simulink model "ddc_bpm_476_066"  (Simulink 7.8)
settings: Solver=ode45  StartTime=0.0  StopTime=2e-3  RelTol=1e-3
undefined symbols (not defined in the file): decim_factor_poly_35, dt_sim, frev_476, Fs_adc, n_ch, n_ovs, R_fofb, R_sec, R_sec_cfir, R_sec_pfir, xlipgetpartsetting
libraries: xbsIndex_r4 x1491, simulink x7
(part 1 of 12)
settings Model: Creator=lucas.russo  LastModifiedBy=lucas.russo
settings HardwareCC: ProdHWDeviceType=ASIC/FPGA->ASIC/FPGA  TargetIntDivRoundTo=Zero  TargetEndianess=LittleEndian  TargetHWDeviceType=MATLAB Host  ProdEqTarget=off

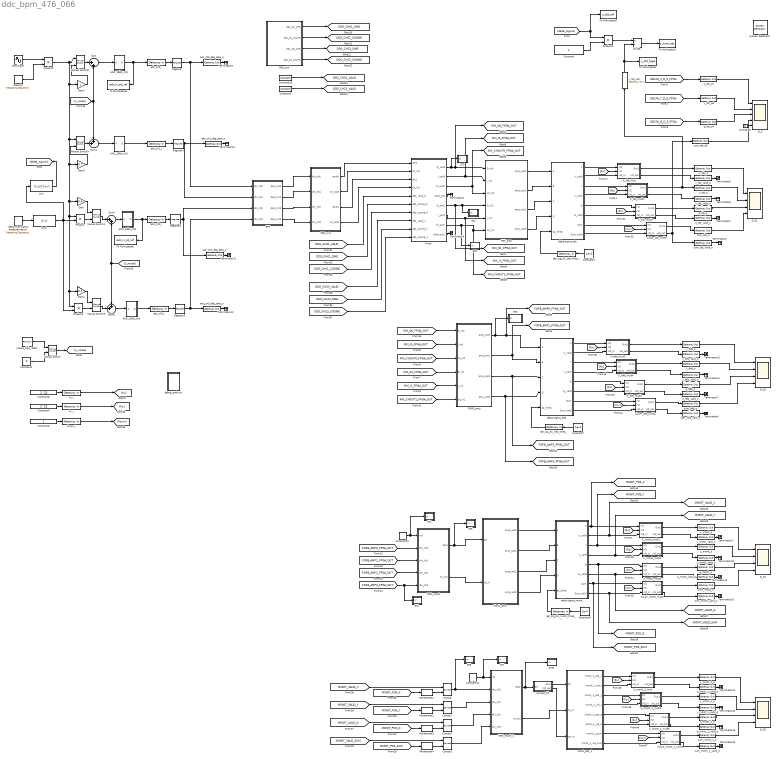
== system ddc_bpm_476_066 ==
  " System Generator" : xbsIndex_r4/ System Generator  Tag=genX  xilinxfamily=artix7  part=xc7a200t  speed=-1  package=ffg1156  synthesis_tool=XST  clock_wrapper=Clock Enables  directory=./netlist_ddc_bpm_476_066_artix7  proj_type=Project Navigator  Synth_file=XST Defaults  Impl_file=ISE Defaults  testbench=off  simulink_period=1/Fs_adc/n_ovs  sysclk_period=1/Fs_adc/n_ovs*1e9  dcm_input_clock_period=10  incr_netlist=off  trim_vbits=Everywhere in SubSystem  dbl_ovrd=According to Block Masks  core_generation=According to Block Masks  run_coregen=off  deprecated_control=off  eval_field=0  block_type=sysgen
  ADC_16bit_ch0 : Subsystem
  ADC_16bit_ch1 : Subsystem
  ADC_16bit_ch2 : Subsystem
  ADC_16bit_ch3 : Subsystem
  BPF : Subsystem
  Concat{,1..3} (4 alike) : xbsIndex_r4/Concat  num_inputs=2  dbl_ovrd=off  block_type=concat
  Constant : Constant
  Constant1 : Constant  Value=1e-4  OutDataTypeStr=fixdt(1,26,22)
  Constant10 : xbsIndex_r4/Constant  const=0  gui_display_data_type=Boolean  arith_type=Boolean  n_bits=16  bin_pt=14  preci_type=Single  exp_width=8  frac_width=24  explicit_period=on  period=(1/Fs_adc*R_fofb)/n_ovs/2  equ=P=C  opselect=C  inp2=PCIN>>17  opr=+  inp1=P  carry=CIN  dbl_ovrd=off  block_type=constant
  Constant11 : xbsIndex_r4/Constant  const=0  gui_display_data_type=Boolean  arith_type=Boolean  n_bits=16  bin_pt=14  preci_type=Single  exp_width=8  frac_width=24  explicit_period=on  period=(1/Fs_adc*R_fofb*R_sec*R_sec_cfir*R_sec_pfir)/n_ovs/2  equ=P=C  opselect=C  inp2=PCIN>>17  opr=+  inp1=P  carry=CIN  dbl_ovrd=off  block_type=constant
  Constant15 : xbsIndex_r4/Constant  const=1  gui_display_data_type=Boolean  arith_type=Boolean  n_bits=24  bin_pt=22  preci_type=Single  exp_width=8  frac_width=24  explicit_period=on  period=1/Fs_adc/n_ovs  equ=P=C  opselect=C  inp2=PCIN>>17  opr=+  inp1=P  carry=CIN  dbl_ovrd=off  block_type=constant
  Constant2 : Constant  Value=0  SampleTime=0
  Constant3 : xbsIndex_r4/Constant  const=1  gui_display_data_type=Boolean  arith_type=Boolean  n_bits=24  bin_pt=22  preci_type=Single  exp_width=8  frac_width=24  explicit_period=on  period=1/Fs_adc/n_ovs  equ=P=C  opselect=C  inp2=PCIN>>17  opr=+  inp1=P  carry=CIN  dbl_ovrd=off  block_type=constant
  Constant4 : Constant  Value=2^23
  Constant5 : Constant  Value=0
  Constant6 : Constant
  Constant7 : Constant  Value=1e-4  OutDataTypeStr=fixdt(1,26,22)
  Constant8 : Constant  Value=2^23
  Constant9 : Constant  Value=1e-4  OutDataTypeStr=fixdt(1,26,22)
  DDS_sub : Subsystem
  D_S : Scope  NumInputPorts=5
      settings: TimeRange=0.0004  YMin=-1~0~10~0~0  YMax=1~0.00025~100~2.5~1  SaveName=ScopeData7  MaxDataPoints=1000000  SampleInput=on
  D_S{1,3..5} (4 alike) : Scope  NumInputPorts=4
      D_S1 settings: TimeRange=0.0003  YMin=-1~-1~-1~0.414326  YMax=1~1~1~0.414329  SaveName=ScopeData6  MaxDataPoints=1000000  SampleInput=on
      D_S3 settings: TimeRange=0.0003  YMin=-1~-1~-1~0.0190031  YMax=1~1~1~0.0210035  SaveName=ScopeData2  MaxDataPoints=1000000  SampleInput=on
      D_S4 settings: TimeRange=0.0003  YMin=-1~-1~-1~0.0190031  YMax=1~1~1~0.0210035  SaveName=ScopeData3  MaxDataPoints=1000000  SampleInput=on
      D_S5 settings: TimeRange=0.0003  YMin=-1~-1~-1~0.0190031  YMax=1~1~1~0.0210035  SaveName=ScopeData20  MaxDataPoints=1000000  SampleInput=on
  Divide : Product  Inputs=*/
  FOFB_amp : Subsystem
  Fcn : Fcn  Expr=(1-u)/(1+u)
  Fcn1 : Fcn  Expr=(1-u)
  Gain : Gain  Gain=0.4
  Gain2 : Gain
  Gain3 : Gain  Gain=0.7
  Gain4 : Gain  Gain=0.1
  K_fofb_mult3 : Subsystem
  K_fofb_mult4 : Subsystem
  K_fofb_mult5 : Subsystem
  K_monit_1_mult : Subsystem
  K_monit_1_mult2 : Subsystem
  K_monit_1_mult6 : Subsystem
  K_monit_mult3 : Subsystem
  K_monit_mult4 : Subsystem
  K_monit_mult5 : Subsystem
  K_tbt_mult : Subsystem
  K_tbt_mult1 : Subsystem
  K_tbt_mult2 : Subsystem
  Ksum_fofb_mult4 : Subsystem
  Ksum_i : xbsIndex_r4/Gateway In  gui_display_data_type=Fixed-point  arith_type="Signed  (2's comp)"  n_bits=25  bin_pt=23  preci_type=Single  exp_width=8  frac_width=24  quantization=Truncate  overflow=Flag as error  period=1/Fs_adc  dbl_ovrd=off  timing_constraint=Data Rate  locs_specified=off  LOCs={}  inherit_from_input=off  UseAsADC=off  ADCChannel='1'  hdl_port=on  block_type=gatewayin
      settings: infoedit="Gateway in block.  Converts inputs of type Simulink integer, single, double and fixed point to  Xilinx fixed-point or floating-point data type.<br><br>Hardware notes:  In hardware these blocks become top level input ports."
  Ksum_monit_1_mult1 : Subsystem
  Ksum_monit_mult2 : Subsystem
  Ksum_tbt_mult3 : Subsystem
  Kx_i : xbsIndex_r4/Gateway In  gui_display_data_type=Fixed-point  arith_type="Signed  (2's comp)"  n_bits=25  bin_pt=0  preci_type=Single  exp_width=8  frac_width=24  quantization=Truncate  overflow=Flag as error  period=1/Fs_adc  dbl_ovrd=off  timing_constraint=Data Rate  locs_specified=off  LOCs={}  inherit_from_input=off  UseAsADC=off  ADCChannel='1'  hdl_port=on  block_type=gatewayin
      settings: infoedit="Gateway in block.  Converts inputs of type Simulink integer, single, double and fixed point to  Xilinx fixed-point or floating-point data type.<br><br>Hardware notes:  In hardware these blocks become top level input ports."
  Ky_i : xbsIndex_r4/Gateway In  gui_display_data_type=Fixed-point  arith_type="Signed  (2's comp)"  n_bits=25  bin_pt=0  preci_type=Single  exp_width=8  frac_width=24  quantization=Truncate  overflow=Flag as error  period=1/Fs_adc  dbl_ovrd=off  timing_constraint=Data Rate  locs_specified=off  LOCs={}  inherit_from_input=off  UseAsADC=off  ADCChannel='1'  hdl_port=on  block_type=gatewayin
      settings: infoedit="Gateway in block.  Converts inputs of type Simulink integer, single, double and fixed point to  Xilinx fixed-point or floating-point data type.<br><br>Hardware notes:  In hardware these blocks become top level input ports."
  Manual Switch : simulink/Signal Routing/Manual Switch  sw=0  action=0  varsize=off
  Manual Switch2 : simulink/Signal Routing/Manual Switch  sw=0  action=0  varsize=off
  Manual Switch3 : simulink/Signal Routing/Manual Switch  sw=0  action=0  varsize=off
  Manual Switch4 : simulink/Signal Routing/Manual Switch  sw=1  action=0  varsize=off
  Manual Switch5 : simulink/Signal Routing/Manual Switch  sw=1  action=0  varsize=off
  Mixer : Subsystem
  Monit_amp : Subsystem
  Product{,1..3} (4 alike) : Product  RndMeth=Zero
  Register{,1..3} (4 alike) : xbsIndex_r4/Register  init=0  rst=off  en=off  dbl_ovrd=off  block_type=register
  Reinterpret{1..4} (4 alike) : xbsIndex_r4/Reinterpret  force_arith_type=on  arith_type=Unsigned  force_bin_pt=on  bin_pt=0  block_type=reinterpret
  ST1 : Subsystem
  ST10 : Subsystem
  ST2 : Subsystem
  ST3 : Subsystem
  ST4 : Subsystem
  ST5 : Subsystem
  ST6 : Subsystem
  ST7 : Subsystem
  ST8 : Subsystem
  ST9 : Subsystem
  Sine Wave : Sin  Frequency=2*pi*frev_476  SampleTime=0
  Sum : Sum  Inputs=|++
  Sum1 : Sum  Inputs=++|
  Sum2 : Sum  Inputs=|++
  Sum3 : Sum  Inputs=++|
  TBT_amp : Subsystem
  TDM_mix : Subsystem
  TDM_monit : Subsystem
  TDM_monit_1 : Subsystem
  Terminator{1..22} (22 alike) : Terminator
  To Workspace1 : ToWorkspace  VariableName=y_tbt_fpga  SampleTime=-1  SaveFormat=Structure With Time
  To Workspace2 : ToWorkspace  VariableName=y_error_tbt  SampleTime=-1  SaveFormat=Structure With Time
  To Workspace3 : ToWorkspace  VariableName=y_tbt_ref  SampleTime=-1  SaveFormat=Structure With Time
  To Workspace4 : ToWorkspace  VariableName=adc_in_ab_ref  SampleTime=-1  SaveFormat=Structure With Time
  To Workspace5 : ToWorkspace  VariableName=adc_in_cd_ref  SampleTime=-1  SaveFormat=Structure With Time
  adc_ch0_dbg_data_o : xbsIndex_r4/Gateway Out  inherit_from_input=on  hdl_port=on  timing_constraint=Data Rate  locs_specified=off  LOCs={}  UseAsDAC=off  DACChannel='1'  block_type=gatewayout
      settings: infoedit="Gateway out block.  Converts Xilinx fixed-point or floating-point type inputs into ouputs of type Simulink integer, single, double, or fixed point.<br><br>Hardware notes:  In hardware these blocks become top level output ports or are discarded, depending on how they are configured."
  adc_ch0_i : xbsIndex_r4/Gateway In  gui_display_data_type=Fixed-point  arith_type="Signed  (2's comp)"  n_bits=16  bin_pt=15  preci_type=Single  exp_width=8  frac_width=24  quantization=Truncate  overflow=Flag as error  period=1/Fs_adc  dbl_ovrd=off  timing_constraint=None  locs_specified=off  LOCs={}  inherit_from_input=off  UseAsADC=off  ADCChannel='1'  hdl_port=on  block_type=gatewayin
      settings: infoedit="Gateway in block.  Converts inputs of type Simulink integer, single, double and fixed point to  Xilinx fixed-point or floating-point data type.<br><br>Hardware notes:  In hardware these blocks become top level input ports."
  adc_ch1_dbg_data_o : xbsIndex_r4/Gateway Out  inherit_from_input=on  hdl_port=on  timing_constraint=Data Rate  locs_specified=off  LOCs={}  UseAsDAC=off  DACChannel='1'  block_type=gatewayout
      settings: infoedit="Gateway out block.  Converts Xilinx fixed-point or floating-point type inputs into ouputs of type Simulink integer, single, double, or fixed point.<br><br>Hardware notes:  In hardware these blocks become top level output ports or are discarded, depending on how they are configured."
  adc_ch1_i : xbsIndex_r4/Gateway In  gui_display_data_type=Fixed-point  arith_type="Signed  (2's comp)"  n_bits=16  bin_pt=15  preci_type=Single  exp_width=8  frac_width=24  quantization=Truncate  overflow=Flag as error  period=1/Fs_adc  dbl_ovrd=off  timing_constraint=None  locs_specified=off  LOCs={}  inherit_from_input=off  UseAsADC=off  ADCChannel='1'  hdl_port=on  block_type=gatewayin
      settings: infoedit="Gateway in block.  Converts inputs of type Simulink integer, single, double and fixed point to  Xilinx fixed-point or floating-point data type.<br><br>Hardware notes:  In hardware these blocks become top level input ports."
  adc_ch2_dbg_data_o : xbsIndex_r4/Gateway Out  inherit_from_input=on  hdl_port=on  timing_constraint=Data Rate  locs_specified=off  LOCs={}  UseAsDAC=off  DACChannel='1'  block_type=gatewayout
      settings: infoedit="Gateway out block.  Converts Xilinx fixed-point or floating-point type inputs into ouputs of type Simulink integer, single, double, or fixed point.<br><br>Hardware notes:  In hardware these blocks become top level output ports or are discarded, depending on how they are configured."
  adc_ch2_i : xbsIndex_r4/Gateway In  gui_display_data_type=Fixed-point  arith_type="Signed  (2's comp)"  n_bits=16  bin_pt=15  preci_type=Single  exp_width=8  frac_width=24  quantization=Truncate  overflow=Flag as error  period=1/Fs_adc  dbl_ovrd=off  timing_constraint=None  locs_specified=off  LOCs={}  inherit_from_input=off  UseAsADC=off  ADCChannel='1'  hdl_port=on  block_type=gatewayin
      settings: infoedit="Gateway in block.  Converts inputs of type Simulink integer, single, double and fixed point to  Xilinx fixed-point or floating-point data type.<br><br>Hardware notes:  In hardware these blocks become top level input ports."
  adc_ch3_dbg_data_o : xbsIndex_r4/Gateway Out  inherit_from_input=on  hdl_port=on  timing_constraint=Data Rate  locs_specified=off  LOCs={}  UseAsDAC=off  DACChannel='1'  block_type=gatewayout
      settings: infoedit="Gateway out block.  Converts Xilinx fixed-point or floating-point type inputs into ouputs of type Simulink integer, single, double, or fixed point.<br><br>Hardware notes:  In hardware these blocks become top level output ports or are discarded, depending on how they are configured."
  adc_ch3_i : xbsIndex_r4/Gateway In  gui_display_data_type=Fixed-point  arith_type="Signed  (2's comp)"  n_bits=16  bin_pt=15  preci_type=Single  exp_width=8  frac_width=24  quantization=Truncate  overflow=Flag as error  period=1/Fs_adc  dbl_ovrd=off  timing_constraint=None  locs_specified=off  LOCs={}  inherit_from_input=off  UseAsADC=off  ADCChannel='1'  hdl_port=on  block_type=gatewayin
      settings: infoedit="Gateway in block.  Converts inputs of type Simulink integer, single, double and fixed point to  Xilinx fixed-point or floating-point data type.<br><br>Hardware notes:  In hardware these blocks become top level input ports."
  convert_filt : Subsystem
  debug_analysis : Subsystem
  del_sig_div_fofb_thres_i : xbsIndex_r4/Gateway In  gui_display_data_type=Fixed-point  arith_type="Signed  (2's comp)"  n_bits=26  bin_pt=22  preci_type=Single  exp_width=8  frac_width=24  quantization=Truncate  overflow=Flag as error  period=1/Fs_adc  dbl_ovrd=off  timing_constraint=Data Rate  locs_specified=off  LOCs={}  inherit_from_input=off  UseAsADC=off  ADCChannel='1'  hdl_port=on  block_type=gatewayin
      settings: infoedit="Gateway in block.  Converts inputs of type Simulink integer, single, double and fixed point to  Xilinx fixed-point or floating-point data type.<br><br>Hardware notes:  In hardware these blocks become top level input ports."
  del_sig_div_monit_thres_i : xbsIndex_r4/Gateway In  gui_display_data_type=Fixed-point  arith_type="Signed  (2's comp)"  n_bits=26  bin_pt=22  preci_type=Single  exp_width=8  frac_width=24  quantization=Truncate  overflow=Flag as error  period=1/Fs_adc  dbl_ovrd=off  timing_constraint=Data Rate  locs_specified=off  LOCs={}  inherit_from_input=off  UseAsADC=off  ADCChannel='1'  hdl_port=on  block_type=gatewayin
      settings: infoedit="Gateway in block.  Converts inputs of type Simulink integer, single, double and fixed point to  Xilinx fixed-point or floating-point data type.<br><br>Hardware notes:  In hardware these blocks become top level input ports."
  del_sig_div_tbt_thres_i : xbsIndex_r4/Gateway In  gui_display_data_type=Fixed-point  arith_type="Signed  (2's comp)"  n_bits=26  bin_pt=22  preci_type=Single  exp_width=8  frac_width=24  quantization=Truncate  overflow=Flag as error  period=1/Fs_adc  dbl_ovrd=off  timing_constraint=Data Rate  locs_specified=off  LOCs={}  inherit_from_input=off  UseAsADC=off  ADCChannel='1'  hdl_port=on  block_type=gatewayin
      settings: infoedit="Gateway in block.  Converts inputs of type Simulink integer, single, double and fixed point to  Xilinx fixed-point or floating-point data type.<br><br>Hardware notes:  In hardware these blocks become top level input ports."
  delta-over-sigma expected result : simulink/Sources/Repeating Sequence  rep_seq_t=[0 0.25e-4 0.25e-4 0.5e-4 0.5e-4 0.75e-4 0.75e-4 1e-4]  rep_seq_y=0.5 * [1 1 1 1 1 1 1 1]
  delta-sigma_fofb : Subsystem
  delta-sigma_monit : Subsystem
  delta-sigma_tbt : Subsystem
  intensity : simulink/Sources/Repeating Sequence  rep_seq_t=[0 1e-4 1e-4 2e-4 2e-4 3e-4 3e-4 4e-4]  rep_seq_y=[1 1 0.1 0.1 0.01 0.01 0.001 0.001]
  monit_pos_1 : Subsystem
  q_fofb_o : xbsIndex_r4/Gateway Out  inherit_from_input=on  hdl_port=on  timing_constraint=None  locs_specified=off  LOCs={}  UseAsDAC=off  DACChannel='1'  block_type=gatewayout
      settings: infoedit="Gateway out block.  Converts Xilinx fixed-point or floating-point type inputs into ouputs of type Simulink integer, single, double, or fixed point.<br><br>Hardware notes:  In hardware these blocks become top level output ports or are discarded, depending on how they are configured."
  q_fofb_valid_o : xbsIndex_r4/Gateway Out  inherit_from_input=on  hdl_port=on  timing_constraint=Data Rate  locs_specified=off  LOCs={}  UseAsDAC=off  DACChannel='1'  block_type=gatewayout
      settings: infoedit="Gateway out block.  Converts Xilinx fixed-point or floating-point type inputs into ouputs of type Simulink integer, single, double, or fixed point.<br><br>Hardware notes:  In hardware these blocks become top level output ports or are discarded, depending on how they are configured."
  q_monit_1_o : xbsIndex_r4/Gateway Out  inherit_from_input=on  hdl_port=on  timing_constraint=None  locs_specified=off  LOCs={}  UseAsDAC=off  DACChannel='1'  block_type=gatewayout
      settings: infoedit="Gateway out block.  Converts Xilinx fixed-point or floating-point type inputs into ouputs of type Simulink integer, single, double, or fixed point.<br><br>Hardware notes:  In hardware these blocks become top level output ports or are discarded, depending on how they are configured."
  q_monit_1_valid_o : xbsIndex_r4/Gateway Out  inherit_from_input=on  hdl_port=on  timing_constraint=Data Rate  locs_specified=off  LOCs={}  UseAsDAC=off  DACChannel='1'  block_type=gatewayout
      settings: infoedit="Gateway out block.  Converts Xilinx fixed-point or floating-point type inputs into ouputs of type Simulink integer, single, double, or fixed point.<br><br>Hardware notes:  In hardware these blocks become top level output ports or are discarded, depending on how they are configured."
  q_monit_o : xbsIndex_r4/Gateway Out  inherit_from_input=on  hdl_port=on  timing_constraint=None  locs_specified=off  LOCs={}  UseAsDAC=off  DACChannel='1'  block_type=gatewayout
      settings: infoedit="Gateway out block.  Converts Xilinx fixed-point or floating-point type inputs into ouputs of type Simulink integer, single, double, or fixed point.<br><br>Hardware notes:  In hardware these blocks become top level output ports or are discarded, depending on how they are configured."
  q_monit_valid_o : xbsIndex_r4/Gateway Out  inherit_from_input=on  hdl_port=on  timing_constraint=Data Rate  locs_specified=off  LOCs={}  UseAsDAC=off  DACChannel='1'  block_type=gatewayout
      settings: infoedit="Gateway out block.  Converts Xilinx fixed-point or floating-point type inputs into ouputs of type Simulink integer, single, double, or fixed point.<br><br>Hardware notes:  In hardware these blocks become top level output ports or are discarded, depending on how they are configured."
  q_tbt_o : xbsIndex_r4/Gateway Out  inherit_from_input=on  hdl_port=on  timing_constraint=Data Rate  locs_specified=off  LOCs={}  UseAsDAC=off  DACChannel='1'  block_type=gatewayout
      settings: infoedit="Gateway out block.  Converts Xilinx fixed-point or floating-point type inputs into ouputs of type Simulink integer, single, double, or fixed point.<br><br>Hardware notes:  In hardware these blocks become top level output ports or are discarded, depending on how they are configured."
  q_tbt_o4 : xbsIndex_r4/Gateway Out  inherit_from_input=on  hdl_port=off  timing_constraint=None  locs_specified=off  LOCs={}  UseAsDAC=off  DACChannel='1'  block_type=gatewayout
      settings: infoedit="Gateway out block.  Converts Xilinx fixed-point or floating-point type inputs into ouputs of type Simulink integer, single, double, or fixed point.<br><br>Hardware notes:  In hardware these blocks become top level output ports or are discarded, depending on how they are configured."
  q_tbt_valid_o : xbsIndex_r4/Gateway Out  inherit_from_input=on  hdl_port=on  timing_constraint=Data Rate  locs_specified=off  LOCs={}  UseAsDAC=off  DACChannel='1'  block_type=gatewayout
      settings: infoedit="Gateway out block.  Converts Xilinx fixed-point or floating-point type inputs into ouputs of type Simulink integer, single, double, or fixed point.<br><br>Hardware notes:  In hardware these blocks become top level output ports or are discarded, depending on how they are configured."
  sum_fofb_o : xbsIndex_r4/Gateway Out  inherit_from_input=on  hdl_port=on  timing_constraint=None  locs_specified=off  LOCs={}  UseAsDAC=off  DACChannel='1'  block_type=gatewayout
      settings: infoedit="Gateway out block.  Converts Xilinx fixed-point or floating-point type inputs into ouputs of type Simulink integer, single, double, or fixed point.<br><br>Hardware notes:  In hardware these blocks become top level output ports or are discarded, depending on how they are configured."
  sum_fofb_valid_o : xbsIndex_r4/Gateway Out  inherit_from_input=on  hdl_port=on  timing_constraint=Data Rate  locs_specified=off  LOCs={}  UseAsDAC=off  DACChannel='1'  block_type=gatewayout
      settings: infoedit="Gateway out block.  Converts Xilinx fixed-point or floating-point type inputs into ouputs of type Simulink integer, single, double, or fixed point.<br><br>Hardware notes:  In hardware these blocks become top level output ports or are discarded, depending on how they are configured."
  sum_monit_1_o : xbsIndex_r4/Gateway Out  inherit_from_input=on  hdl_port=on  timing_constraint=None  locs_specified=off  LOCs={}  UseAsDAC=off  DACChannel='1'  block_type=gatewayout
      settings: infoedit="Gateway out block.  Converts Xilinx fixed-point or floating-point type inputs into ouputs of type Simulink integer, single, double, or fixed point.<br><br>Hardware notes:  In hardware these blocks become top level output ports or are discarded, depending on how they are configured."
  sum_monit_1_valid_o : xbsIndex_r4/Gateway Out  inherit_from_input=on  hdl_port=on  timing_constraint=Data Rate  locs_specified=off  LOCs={}  UseAsDAC=off  DACChannel='1'  block_type=gatewayout
      settings: infoedit="Gateway out block.  Converts Xilinx fixed-point or floating-point type inputs into ouputs of type Simulink integer, single, double, or fixed point.<br><br>Hardware notes:  In hardware these blocks become top level output ports or are discarded, depending on how they are configured."
  sum_monit_o : xbsIndex_r4/Gateway Out  inherit_from_input=on  hdl_port=on  timing_constraint=None  locs_specified=off  LOCs={}  UseAsDAC=off  DACChannel='1'  block_type=gatewayout
      settings: infoedit="Gateway out block.  Converts Xilinx fixed-point or floating-point type inputs into ouputs of type Simulink integer, single, double, or fixed point.<br><br>Hardware notes:  In hardware these blocks become top level output ports or are discarded, depending on how they are configured."
  sum_monit_valid_o : xbsIndex_r4/Gateway Out  inherit_from_input=on  hdl_port=on  timing_constraint=Data Rate  locs_specified=off  LOCs={}  UseAsDAC=off  DACChannel='1'  block_type=gatewayout
      settings: infoedit="Gateway out block.  Converts Xilinx fixed-point or floating-point type inputs into ouputs of type Simulink integer, single, double, or fixed point.<br><br>Hardware notes:  In hardware these blocks become top level output ports or are discarded, depending on how they are configured."
  sum_tbt_o : xbsIndex_r4/Gateway Out  inherit_from_input=on  hdl_port=on  timing_constraint=Data Rate  locs_specified=off  LOCs={}  UseAsDAC=off  DACChannel='1'  block_type=gatewayout
      settings: infoedit="Gateway out block.  Converts Xilinx fixed-point or floating-point type inputs into ouputs of type Simulink integer, single, double, or fixed point.<br><br>Hardware notes:  In hardware these blocks become top level output ports or are discarded, depending on how they are configured."
  sum_tbt_o5 : xbsIndex_r4/Gateway Out  inherit_from_input=on  hdl_port=off  timing_constraint=None  locs_specified=off  LOCs={}  UseAsDAC=off  DACChannel='1'  block_type=gatewayout
      settings: infoedit="Gateway out block.  Converts Xilinx fixed-point or floating-point type inputs into ouputs of type Simulink integer, single, double, or fixed point.<br><br>Hardware notes:  In hardware these blocks become top level output ports or are discarded, depending on how they are configured."
  sum_tbt_valid_o : xbsIndex_r4/Gateway Out  inherit_from_input=on  hdl_port=on  timing_constraint=Data Rate  locs_specified=off  LOCs={}  UseAsDAC=off  DACChannel='1'  block_type=gatewayout
      settings: infoedit="Gateway out block.  Converts Xilinx fixed-point or floating-point type inputs into ouputs of type Simulink integer, single, double, or fixed point.<br><br>Hardware notes:  In hardware these blocks become top level output ports or are discarded, depending on how they are configured."
  unoise_1lsb_ 16bit : UniformRandomNumber  Minimum=-0.5*(2/2^16)  Maximum=0.5*(2/2^16)  Seed=49728613  SampleTime=0
  x_fofb_o : xbsIndex_r4/Gateway Out  inherit_from_input=on  hdl_port=on  timing_constraint=None  locs_specified=off  LOCs={}  UseAsDAC=off  DACChannel='1'  block_type=gatewayout
      settings: infoedit="Gateway out block.  Converts Xilinx fixed-point or floating-point type inputs into ouputs of type Simulink integer, single, double, or fixed point.<br><br>Hardware notes:  In hardware these blocks become top level output ports or are discarded, depending on how they are configured."
  x_fofb_valid_o : xbsIndex_r4/Gateway Out  inherit_from_input=on  hdl_port=on  timing_constraint=Data Rate  locs_specified=off  LOCs={}  UseAsDAC=off  DACChannel='1'  block_type=gatewayout
      settings: infoedit="Gateway out block.  Converts Xilinx fixed-point or floating-point type inputs into ouputs of type Simulink integer, single, double, or fixed point.<br><br>Hardware notes:  In hardware these blocks become top level output ports or are discarded, depending on how they are configured."
  x_monit_1_o : xbsIndex_r4/Gateway Out  inherit_from_input=on  hdl_port=on  timing_constraint=None  locs_specified=off  LOCs={}  UseAsDAC=off  DACChannel='1'  block_type=gatewayout
      settings: infoedit="Gateway out block.  Converts Xilinx fixed-point or floating-point type inputs into ouputs of type Simulink integer, single, double, or fixed point.<br><br>Hardware notes:  In hardware these blocks become top level output ports or are discarded, depending on how they are configured."
  x_monit_1_valid_o : xbsIndex_r4/Gateway Out  inherit_from_input=on  hdl_port=on  timing_constraint=Data Rate  locs_specified=off  LOCs={}  UseAsDAC=off  DACChannel='1'  block_type=gatewayout
      settings: infoedit="Gateway out block.  Converts Xilinx fixed-point or floating-point type inputs into ouputs of type Simulink integer, single, double, or fixed point.<br><br>Hardware notes:  In hardware these blocks become top level output ports or are discarded, depending on how they are configured."
  x_monit_o : xbsIndex_r4/Gateway Out  inherit_from_input=on  hdl_port=on  timing_constraint=None  locs_specified=off  LOCs={}  UseAsDAC=off  DACChannel='1'  block_type=gatewayout
      settings: infoedit="Gateway out block.  Converts Xilinx fixed-point or floating-point type inputs into ouputs of type Simulink integer, single, double, or fixed point.<br><br>Hardware notes:  In hardware these blocks become top level output ports or are discarded, depending on how they are configured."
  x_monit_valid_o : xbsIndex_r4/Gateway Out  inherit_from_input=on  hdl_port=on  timing_constraint=Data Rate  locs_specified=off  LOCs={}  UseAsDAC=off  DACChannel='1'  block_type=gatewayout
      settings: infoedit="Gateway out block.  Converts Xilinx fixed-point or floating-point type inputs into ouputs of type Simulink integer, single, double, or fixed point.<br><br>Hardware notes:  In hardware these blocks become top level output ports or are discarded, depending on how they are configured."
  x_tbt_o : xbsIndex_r4/Gateway Out  inherit_from_input=on  hdl_port=on  timing_constraint=Data Rate  locs_specified=off  LOCs={}  UseAsDAC=off  DACChannel='1'  block_type=gatewayout
      settings: infoedit="Gateway out block.  Converts Xilinx fixed-point or floating-point type inputs into ouputs of type Simulink integer, single, double, or fixed point.<br><br>Hardware notes:  In hardware these blocks become top level output ports or are discarded, depending on how they are configured."
  x_tbt_o1 : xbsIndex_r4/Gateway Out  inherit_from_input=on  hdl_port=off  timing_constraint=None  locs_specified=off  LOCs={}  UseAsDAC=off  DACChannel='1'  block_type=gatewayout
      settings: infoedit="Gateway out block.  Converts Xilinx fixed-point or floating-point type inputs into ouputs of type Simulink integer, single, double, or fixed point.<br><br>Hardware notes:  In hardware these blocks become top level output ports or are discarded, depending on how they are configured."
  x_tbt_valid_o : xbsIndex_r4/Gateway Out  inherit_from_input=on  hdl_port=on  timing_constraint=Data Rate  locs_specified=off  LOCs={}  UseAsDAC=off  DACChannel='1'  block_type=gatewayout
      settings: infoedit="Gateway out block.  Converts Xilinx fixed-point or floating-point type inputs into ouputs of type Simulink integer, single, double, or fixed point.<br><br>Hardware notes:  In hardware these blocks become top level output ports or are discarded, depending on how they are configured."
  y_fofb_o : xbsIndex_r4/Gateway Out  inherit_from_input=on  hdl_port=on  timing_constraint=None  locs_specified=off  LOCs={}  UseAsDAC=off  DACChannel='1'  block_type=gatewayout
      settings: infoedit="Gateway out block.  Converts Xilinx fixed-point or floating-point type inputs into ouputs of type Simulink integer, single, double, or fixed point.<br><br>Hardware notes:  In hardware these blocks become top level output ports or are discarded, depending on how they are configured."
  y_fofb_valid_o : xbsIndex_r4/Gateway Out  inherit_from_input=on  hdl_port=on  timing_constraint=Data Rate  locs_specified=off  LOCs={}  UseAsDAC=off  DACChannel='1'  block_type=gatewayout
      settings: infoedit="Gateway out block.  Converts Xilinx fixed-point or floating-point type inputs into ouputs of type Simulink integer, single, double, or fixed point.<br><br>Hardware notes:  In hardware these blocks become top level output ports or are discarded, depending on how they are configured."
  y_monit_1_o : xbsIndex_r4/Gateway Out  inherit_from_input=on  hdl_port=on  timing_constraint=None  locs_specified=off  LOCs={}  UseAsDAC=off  DACChannel='1'  block_type=gatewayout
      settings: infoedit="Gateway out block.  Converts Xilinx fixed-point or floating-point type inputs into ouputs of type Simulink integer, single, double, or fixed point.<br><br>Hardware notes:  In hardware these blocks become top level output ports or are discarded, depending on how they are configured."
  y_monit_1_valid_o : xbsIndex_r4/Gateway Out  inherit_from_input=on  hdl_port=on  timing_constraint=Data Rate  locs_specified=off  LOCs={}  UseAsDAC=off  DACChannel='1'  block_type=gatewayout
      settings: infoedit="Gateway out block.  Converts Xilinx fixed-point or floating-point type inputs into ouputs of type Simulink integer, single, double, or fixed point.<br><br>Hardware notes:  In hardware these blocks become top level output ports or are discarded, depending on how they are configured."
  y_monit_o : xbsIndex_r4/Gateway Out  inherit_from_input=on  hdl_port=on  timing_constraint=None  locs_specified=off  LOCs={}  UseAsDAC=off  DACChannel='1'  block_type=gatewayout
      settings: infoedit="Gateway out block.  Converts Xilinx fixed-point or floating-point type inputs into ouputs of type Simulink integer, single, double, or fixed point.<br><br>Hardware notes:  In hardware these blocks become top level output ports or are discarded, depending on how they are configured."
  y_monit_valid_o : xbsIndex_r4/Gateway Out  inherit_from_input=on  hdl_port=on  timing_constraint=Data Rate  locs_specified=off  LOCs={}  UseAsDAC=off  DACChannel='1'  block_type=gatewayout
      settings: infoedit="Gateway out block.  Converts Xilinx fixed-point or floating-point type inputs into ouputs of type Simulink integer, single, double, or fixed point.<br><br>Hardware notes:  In hardware these blocks become top level output ports or are discarded, depending on how they are configured."
  y_tbt_o : xbsIndex_r4/Gateway Out  inherit_from_input=on  hdl_port=on  timing_constraint=Data Rate  locs_specified=off  LOCs={}  UseAsDAC=off  DACChannel='1'  block_type=gatewayout
      settings: infoedit="Gateway out block.  Converts Xilinx fixed-point or floating-point type inputs into ouputs of type Simulink integer, single, double, or fixed point.<br><br>Hardware notes:  In hardware these blocks become top level output ports or are discarded, depending on how they are configured."
  y_tbt_o6 : xbsIndex_r4/Gateway Out  inherit_from_input=on  hdl_port=off  timing_constraint=None  locs_specified=off  LOCs={}  UseAsDAC=off  DACChannel='1'  block_type=gatewayout
      settings: infoedit="Gateway out block.  Converts Xilinx fixed-point or floating-point type inputs into ouputs of type Simulink integer, single, double, or fixed point.<br><br>Hardware notes:  In hardware these blocks become top level output ports or are discarded, depending on how they are configured."
  y_tbt_out : xbsIndex_r4/Gateway Out  inherit_from_input=on  hdl_port=off  timing_constraint=None  locs_specified=off  LOCs={}  UseAsDAC=off  DACChannel='1'  block_type=gatewayout
      settings: infoedit="Gateway out block.  Converts Xilinx fixed-point or floating-point type inputs into ouputs of type Simulink integer, single, double, or fixed point.<br><br>Hardware notes:  In hardware these blocks become top level output ports or are discarded, depending on how they are configured."
  y_tbt_valid_o : xbsIndex_r4/Gateway Out  inherit_from_input=on  hdl_port=on  timing_constraint=Data Rate  locs_specified=off  LOCs={}  UseAsDAC=off  DACChannel='1'  block_type=gatewayout
      settings: infoedit="Gateway out block.  Converts Xilinx fixed-point or floating-point type inputs into ouputs of type Simulink integer, single, double, or fixed point.<br><br>Hardware notes:  In hardware these blocks become top level output ports or are discarded, depending on how they are configured."
  tag scope: DDS_CH01_COSINE=global, DDS_CH01_SINE=global, DDS_CH01_VALID=global, DDS_CH23_COSINE=global, DDS_CH23_SINE=global, DDS_CH23_VALID=global, FOFB_AMP0_FPGA_OUT=global, FOFB_AMP1_FPGA_OUT=global, FOFB_AMP2_FPGA_OUT=global, FOFB_AMP3_FPGA_OUT=global, MIX_CHOUT0_FPGA_OUT=global, MIX_CHOUT1_FPGA_OUT=global, MIX_I0_FPGA_OUT=global, MIX_I1_FPGA_OUT=global, MIX_Q0_FPGA_OUT=global, MIX_Q1_FPGA_OUT=global, MONIT_POS_Q=global, MONIT_POS_SUM=global, MONIT_POS_X=global, MONIT_POS_Y=global, MONIT_VALID_Q=global, MONIT_VALID_SUM=global, MONIT_VALID_X=global, MONIT_VALID_Y=global
  wires:
  delta-over-sigma expected result/1 -> Fcn1/1
  Fcn/1 -> [delta_sigma]
  ADC_16bit_ch0/1(D) -> To Workspace4/1, adc_ch0_i/1
  ADC_16bit_ch1/1(D) -> adc_ch1_i/1
  ADC_16bit_ch2/1(D) -> To Workspace5/1, adc_ch2_i/1
  ADC_16bit_ch3/1(D) -> adc_ch3_i/1
  Constant/1 -> Product3/2
  Product3/1 -> Divide/1
  Divide/1 -> To Workspace2/1
  [delta_sigma] -> Product3/1, To Workspace3/1
  [DELTA_X_D_S_FPGA] -> x_tbt_o1/1
  [DELTA_Y_D_S_FPGA] -> y_tbt_o6/1
  [DELTA_Q_D_S_FPGA] -> q_tbt_o4/1
  x_tbt_o1/1 -> D_S/1
  y_tbt_o6/1 -> D_S/2
  q_tbt_o4/1 -> D_S/3
  sum_tbt_o5/1 -> D_S/4
  x_tbt_o/1 -> D_S1/1
  y_tbt_o/1 -> D_S1/2
  q_tbt_o/1 -> D_S1/3
  sum_tbt_o/1 -> D_S1/4
  y_tbt_out/1 -> Divide/2, To Workspace1/1
  del_sig_div_tbt_thres_i/1 -> delta-sigma_tbt/5(ds_thres)
  Fcn1/1 -> Product/2, Product1/2, Fcn/1
  Constant1/1 -> del_sig_div_tbt_thres_i/1
  intensity/1 -> Product2/2
  Sine Wave/1 -> Product2/1
  Product2/1 -> Manual Switch2/1, Gain2/1, Manual Switch3/1, Gain3/1, Product/1, Product1/1, Gain4/1, Gain/1
  Sum/1 -> ADC_16bit_ch0/1(A)
  Sum1/1 -> ADC_16bit_ch1/1(A)
  Sum2/1 -> ADC_16bit_ch2/1(A)
  Sum3/1 -> ADC_16bit_ch3/1(A)
  unoise_1lsb_ 16bit/1 -> Manual Switch/1
  Constant2/1 -> Manual Switch/2
  Manual Switch/1 -> [u_noise]
  [u_noise] -> Sum/2, Sum1/1
  [u_noise] -> Sum2/2, Sum3/1
  Constant5/1 -> D_S/5
  Ksum_tbt_mult3/1(Out1) -> sum_tbt_o/1
  Constant6/1 -> Ksum_i/1
  Constant8/1 -> Kx_i/1
  Constant4/1 -> Ky_i/1
  Kx_i/1 -> [Kx]
  Ky_i/1 -> [Ky]
  Ksum_i/1 -> [Ksum]
  adc_ch0_i/1 -> Register/1
  adc_ch1_i/1 -> Register1/1
  adc_ch2_i/1 -> Register2/1
  adc_ch3_i/1 -> Register3/1
  [DDS_CH01_VALID] -> Mixer/5(dds_valid_0)
  [DDS_CH01_COSINE] -> Mixer/7(dds_cosine_0)
  [DDS_CH01_SINE] -> Mixer/6(dds_msine_0)
  adc_ch0_dbg_data_o/1 -> Terminator9/1
  adc_ch1_dbg_data_o/1 -> Terminator10/1
  adc_ch2_dbg_data_o/1 -> Terminator11/1
  adc_ch3_dbg_data_o/1 -> Terminator12/1
  TDM_mix/2(ch_out0) -> Mixer/2(ch_in0)
  TDM_mix/3(dout1) -> Mixer/3(din1)
  TDM_mix/4(ch_out1) -> Mixer/4(ch_in1)
  BPF/1(dout_ch0) -> TDM_mix/1(din_ch0)
  BPF/2(dout_ch1) -> TDM_mix/2(din_ch1)
  BPF/3(dout_ch2) -> TDM_mix/3(din_ch2)
  TDM_mix/1(dout0) -> Mixer/1(din0)
  Mixer/1(Q_out0) -> [MIX_Q0_FPGA_OUT], TBT_amp/1(Q_in0), ST3/1(In)
  Mixer/2(I_out0) -> TBT_amp/2(I_in0), [MIX_I0_FPGA_OUT]
  Mixer/3(ch_out0) -> TBT_amp/3(ch_in0), [MIX_CHOUT0_FPGA_OUT]
  Mixer/5(Q_out1) -> [MIX_Q1_FPGA_OUT], TBT_amp/4(Q_in1), ST4/1(In)
  Mixer/6(I_out1) -> TBT_amp/5(I_in1), [MIX_I1_FPGA_OUT]
  Mixer/7(ch_out1) -> TBT_amp/6(ch_in1), [MIX_CHOUT1_FPGA_OUT], ST6/1(In)
  Mixer/4(valid_out) -> Terminator1/1
  Mixer/8(valid_out1) -> Terminator4/1
  TBT_amp/1(amp_out0) -> delta-sigma_tbt/1(A)
  TBT_amp/2(amp_out1) -> delta-sigma_tbt/2(B)
  TBT_amp/3(amp_out2) -> delta-sigma_tbt/3(C)
  TBT_amp/4(amp_out3) -> delta-sigma_tbt/4(D)
  del_sig_div_fofb_thres_i/1 -> delta-sigma_fofb/5(ds_thres)
  Constant7/1 -> del_sig_div_fofb_thres_i/1
  x_fofb_o/1 -> D_S3/1
  y_fofb_o/1 -> D_S3/2
  q_fofb_o/1 -> D_S3/3
  sum_fofb_o/1 -> D_S3/4
  FOFB_amp/1(amp_out0) -> [FOFB_AMP0_FPGA_OUT], delta-sigma_fofb/1(A), ST8/1(In)
  FOFB_amp/2(amp_out1) -> [FOFB_AMP1_FPGA_OUT], delta-sigma_fofb/2(B)
  FOFB_amp/3(amp_out2) -> [FOFB_AMP2_FPGA_OUT], delta-sigma_fofb/3(C)
  FOFB_amp/4(amp_out3) -> [FOFB_AMP3_FPGA_OUT], delta-sigma_fofb/4(D)
  [MIX_Q0_FPGA_OUT] -> FOFB_amp/1(Q_in0)
  [MIX_I0_FPGA_OUT] -> FOFB_amp/2(I_in0)
  [MIX_CHOUT0_FPGA_OUT] -> FOFB_amp/3(ch_in0)
  [MIX_Q1_FPGA_OUT] -> FOFB_amp/4(Q_in1)
  [MIX_I1_FPGA_OUT] -> FOFB_amp/5(I_in1)
  [MIX_CHOUT1_FPGA_OUT] -> FOFB_amp/6(ch_in1)
  x_monit_o/1 -> D_S4/1
  sum_monit_o/1 -> D_S4/4
  y_monit_o/1 -> D_S4/2
  q_monit_o/1 -> D_S4/3
  Monit_amp/1(amp_out0) -> delta-sigma_monit/1(A)
  Monit_amp/2(amp_out1) -> delta-sigma_monit/2(B)
  Monit_amp/3(amp_out2) -> delta-sigma_monit/3(C)
  Monit_amp/4(amp_out3) -> delta-sigma_monit/4(D)
  Constant10/1 -> ST1/1(In), TDM_monit/1(rst)
  [FOFB_AMP0_FPGA_OUT] -> TDM_monit/2(din_ch0)
  [FOFB_AMP1_FPGA_OUT] -> TDM_monit/3(din_ch1)
  [FOFB_AMP2_FPGA_OUT] -> TDM_monit/4(din_ch2)
  [FOFB_AMP3_FPGA_OUT] -> ST2/1(In), TDM_monit/5(din_ch3)
  Constant9/1 -> del_sig_div_monit_thres_i/1
  TDM_monit/1(dout) -> Monit_amp/1(din), ST5/1(In)
  TDM_monit/2(ch_out) -> Monit_amp/2(ch_in)
  Register/1 -> adc_ch0_dbg_data_o/1, BPF/1(din_ch0)
  Register1/1 -> adc_ch1_dbg_data_o/1, BPF/2(din_ch1)
  Register2/1 -> adc_ch2_dbg_data_o/1, BPF/3(din_ch2)
  Register3/1 -> adc_ch3_dbg_data_o/1, BPF/4(din_ch3)
  Manual Switch2/1 -> Sum/1
  Gain2/1 -> Manual Switch2/2
  Manual Switch3/1 -> Sum1/2
  Gain3/1 -> Manual Switch3/2
  Gain/1 -> Manual Switch4/1
  Product/1 -> Manual Switch4/2
  Manual Switch4/1 -> Sum2/1
  Gain4/1 -> Manual Switch5/1
  Manual Switch5/1 -> Sum3/2
  Product1/1 -> Manual Switch5/2
  x_monit_1_o/1 -> D_S5/1
  sum_monit_1_o/1 -> D_S5/4
  y_monit_1_o/1 -> D_S5/2
  q_monit_1_o/1 -> D_S5/3
  TDM_monit_1/1(dout) -> ST10/1(In), convert_filt/1(din)
  TDM_monit_1/2(ch_out) -> monit_pos_1/2(ch_in)
  Constant11/1 -> ST7/1(In), TDM_monit_1/1(rst)
  [DDS_CH23_VALID] -> Mixer/8(dds_valid_1)
  [DDS_CH23_SINE] -> Mixer/9(dds_msine_1)
  [DDS_CH23_COSINE] -> Mixer/10(dds_cosine_1)
  DDS_sub/1(dds_01_sine) -> [DDS_CH01_SINE]
  DDS_sub/2(dds_01_cosine) -> [DDS_CH01_COSINE]
  DDS_sub/3(dds_23_sine) -> [DDS_CH23_SINE]
  DDS_sub/4(dds_23_cosine) -> [DDS_CH23_COSINE]
  Constant15/1 -> [DDS_CH01_VALID]
  Constant3/1 -> [DDS_CH23_VALID]
  K_tbt_mult2/1(Out1) -> q_tbt_o/1
  [Kx] -> K_tbt_mult/2(In2)
  [Kx] -> K_tbt_mult2/2(In2)
  [Ksum] -> Ksum_tbt_mult3/2(In2)
  [Ky] -> K_tbt_mult1/2(In2)
  delta-sigma_tbt/1(X) -> K_tbt_mult/1(In1)
  delta-sigma_tbt/2(X_valid) -> K_tbt_mult/3(vld_in)
  delta-sigma_tbt/3(Y) -> K_tbt_mult1/1(In1)
  delta-sigma_tbt/4(Y_valid) -> K_tbt_mult1/3(vld_in)
  delta-sigma_tbt/5(Q) -> K_tbt_mult2/1(In1)
  delta-sigma_tbt/6(Q_valid) -> K_tbt_mult2/3(vld_in)
  delta-sigma_tbt/7(Sum) -> Ksum_tbt_mult3/1(In1)
  delta-sigma_tbt/8(Sum_valid) -> Ksum_tbt_mult3/3(vld_in)
  K_tbt_mult/1(Out1) -> x_tbt_o/1
  K_tbt_mult1/1(Out1) -> y_tbt_o/1, y_tbt_out/1
  q_tbt_valid_o/1 -> Terminator2/1
  sum_tbt_valid_o/1 -> Terminator3/1
  x_tbt_valid_o/1 -> Terminator5/1
  y_tbt_valid_o/1 -> Terminator6/1
  K_tbt_mult/2(vld_out) -> x_tbt_valid_o/1
  K_tbt_mult1/2(vld_out) -> y_tbt_valid_o/1
  K_tbt_mult2/2(vld_out) -> q_tbt_valid_o/1
  Ksum_tbt_mult3/2(vld_out) -> sum_tbt_valid_o/1, sum_tbt_o5/1
  K_fofb_mult5/1(Out1) -> q_fofb_o/1
  [Kx] -> K_fofb_mult3/2(In2)
  [Kx] -> K_fofb_mult5/2(In2)
  [Ksum] -> Ksum_fofb_mult4/2(In2)
  [Ky] -> K_fofb_mult4/2(In2)
  delta-sigma_fofb/1(X) -> K_fofb_mult3/1(In1)
  delta-sigma_fofb/2(X_valid) -> K_fofb_mult3/3(vld_in)
  delta-sigma_fofb/3(Y) -> K_fofb_mult4/1(In1)
  delta-sigma_fofb/4(Y_valid) -> K_fofb_mult4/3(vld_in)
  delta-sigma_fofb/5(Q) -> K_fofb_mult5/1(In1)
  delta-sigma_fofb/6(Q_valid) -> K_fofb_mult5/3(vld_in)
  delta-sigma_fofb/7(Sum) -> Ksum_fofb_mult4/1(In1)
  delta-sigma_fofb/8(Sum_valid) -> Ksum_fofb_mult4/3(vld_in)
  K_fofb_mult3/1(Out1) -> x_fofb_o/1
  K_fofb_mult4/1(Out1) -> y_fofb_o/1
  K_fofb_mult3/2(vld_out) -> x_fofb_valid_o/1
  K_fofb_mult4/2(vld_out) -> y_fofb_valid_o/1
  K_fofb_mult5/2(vld_out) -> q_fofb_valid_o/1
  Ksum_fofb_mult4/1(Out1) -> sum_fofb_o/1
  q_fofb_valid_o/1 -> Terminator7/1
  sum_fofb_valid_o/1 -> Terminator8/1
  x_fofb_valid_o/1 -> Terminator13/1
  y_fofb_valid_o/1 -> Terminator14/1
  Ksum_fofb_mult4/2(vld_out) -> sum_fofb_valid_o/1
  del_sig_div_monit_thres_i/1 -> delta-sigma_monit/5(ds_thres)
  Ksum_monit_mult2/1(Out1) -> sum_monit_o/1
  K_monit_mult5/1(Out1) -> q_monit_o/1
  [Kx] -> K_monit_mult3/2(In2)
  [Kx] -> K_monit_mult5/2(In2)
  [Ksum] -> Ksum_monit_mult2/2(In2)
  [Ky] -> K_monit_mult4/2(In2)
  delta-sigma_monit/1(X) -> K_monit_mult3/1(In1), [MONIT_POS_X]
  delta-sigma_monit/2(X_valid) -> K_monit_mult3/3(vld_in), [MONIT_VALID_X]
  delta-sigma_monit/3(Y) -> K_monit_mult4/1(In1), [MONIT_POS_Y]
  delta-sigma_monit/4(Y_valid) -> K_monit_mult4/3(vld_in), [MONIT_VALID_Y]
  delta-sigma_monit/5(Q) -> K_monit_mult5/1(In1), [MONIT_POS_Q]
  delta-sigma_monit/6(Q_valid) -> K_monit_mult5/3(vld_in), [MONIT_VALID_Q]
  delta-sigma_monit/7(Sum) -> Ksum_monit_mult2/1(In1), [MONIT_POS_SUM]
  delta-sigma_monit/8(Sum_valid) -> Ksum_monit_mult2/3(vld_in), [MONIT_VALID_SUM]
  K_monit_mult3/1(Out1) -> x_monit_o/1
  K_monit_mult4/1(Out1) -> y_monit_o/1
  K_monit_mult3/2(vld_out) -> x_monit_valid_o/1
  K_monit_mult4/2(vld_out) -> y_monit_valid_o/1
  K_monit_mult5/2(vld_out) -> q_monit_valid_o/1
  Ksum_monit_mult2/2(vld_out) -> sum_monit_valid_o/1
  q_monit_valid_o/1 -> Terminator15/1
  sum_monit_valid_o/1 -> Terminator16/1
  x_monit_valid_o/1 -> Terminator17/1
  y_monit_valid_o/1 -> Terminator18/1
  [MONIT_POS_X] -> Reinterpret1/1
  [MONIT_VALID_X] -> Concat/1
  [MONIT_POS_Y] -> Reinterpret2/1
  [MONIT_POS_Q] -> Reinterpret3/1
  [MONIT_POS_SUM] -> Reinterpret4/1
  [MONIT_VALID_Y] -> Concat1/1
  [MONIT_VALID_Q] -> Concat2/1
  [MONIT_VALID_SUM] -> Concat3/1
  Reinterpret1/1 -> Concat/2
  Reinterpret2/1 -> Concat1/2
  Reinterpret4/1 -> Concat3/2
  Concat3/1 -> TDM_monit_1/5(din_ch3)
  Concat/1 -> TDM_monit_1/2(din_ch0), ST9/1(In)
  Concat1/1 -> TDM_monit_1/3(din_ch1)
  Concat2/1 -> TDM_monit_1/4(din_ch2)
  convert_filt/1(dout) -> monit_pos_1/1(din)
  convert_filt/2(vld_out) -> monit_pos_1/3(usr_in)
  K_monit_1_mult6/1(Out1) -> q_monit_1_o/1
  [Kx] -> K_monit_1_mult/2(In2)
  [Kx] -> K_monit_1_mult6/2(In2)
  [Ksum] -> Ksum_monit_1_mult1/2(In2)
  [Ky] -> K_monit_1_mult2/2(In2)
  monit_pos_1/1(monit_1_pos_x) -> K_monit_1_mult/1(In1)
  monit_pos_1/2(monit_1_vld_x) -> K_monit_1_mult/3(vld_in)
  monit_pos_1/3(monit_1_pos_y) -> K_monit_1_mult2/1(In1)
  monit_pos_1/4(monit_1_vld_y) -> K_monit_1_mult2/3(vld_in)
  monit_pos_1/5(monit_1_pos_q) -> K_monit_1_mult6/1(In1)
  monit_pos_1/6(monit_1_vld_q) -> K_monit_1_mult6/3(vld_in)
  monit_pos_1/7(monit_1_sum) -> Ksum_monit_1_mult1/1(In1)
  monit_pos_1/8(monit_1_vld_sum) -> Ksum_monit_1_mult1/3(vld_in)
  K_monit_1_mult/1(Out1) -> x_monit_1_o/1
  K_monit_1_mult2/1(Out1) -> y_monit_1_o/1
  K_monit_1_mult/2(vld_out) -> x_monit_1_valid_o/1
  K_monit_1_mult2/2(vld_out) -> y_monit_1_valid_o/1
  K_monit_1_mult6/2(vld_out) -> q_monit_1_valid_o/1
  Ksum_monit_1_mult1/1(Out1) -> sum_monit_1_o/1
  Ksum_monit_1_mult1/2(vld_out) -> sum_monit_1_valid_o/1
  q_monit_1_valid_o/1 -> Terminator19/1
  sum_monit_1_valid_o/1 -> Terminator20/1
  x_monit_1_valid_o/1 -> Terminator21/1
  y_monit_1_valid_o/1 -> Terminator22/1
  Reinterpret3/1 -> Concat2/2
  BPF/4(dout_ch3) -> TDM_mix/4(din_ch3)

== system ddc_bpm_476_066/ADC_16bit_ch0 ==
  A : Inport  OutDataTypeStr=double
  Conversion3 : DataTypeConversion  OutDataTypeStr=fixdt(1,16,2/2^16/1,0/1)  ConvertRealWorld=Stored Integer (SI)  LockScale=on
  Quantizer : Quantizer  QuantizationInterval=1  SampleTime=dt_sim
  Sampler : ZeroOrderHold  SampleTime=1/Fs_adc
  Saturation : Saturate  UpperLimit=65536/2-1  LowerLimit=-65536/2  OutDataTypeStr=Inherit: Inherit via back propagation
  scale : Gain  Gain=2^16/2  SaturateOnIntegerOverflow=on  OutDataTypeStr=Inherit: Same as input  ParamDataTypeStr=Inherit: Same as input
  D : Outport
  wires:
  A/1 -> scale/1
  Conversion3/1 -> D/1
  Quantizer/1 -> Saturation/1
  Sampler/1 -> Quantizer/1
  Saturation/1 -> Conversion3/1
  scale/1 -> Sampler/1

== system ddc_bpm_476_066/ADC_16bit_ch1 ==
  A : Inport  OutDataTypeStr=double
  Conversion3 : DataTypeConversion  OutDataTypeStr=fixdt(1,16,2/2^16/1,0/1)  ConvertRealWorld=Stored Integer (SI)  LockScale=on
  Quantizer : Quantizer  QuantizationInterval=1  SampleTime=dt_sim
  Sampler : ZeroOrderHold  SampleTime=1/Fs_adc
  Saturation : Saturate  UpperLimit=65536/2-1  LowerLimit=-65536/2  OutDataTypeStr=Inherit: Inherit via back propagation
  scale : Gain  Gain=2^16/2  SaturateOnIntegerOverflow=on  OutDataTypeStr=Inherit: Same as input  ParamDataTypeStr=Inherit: Same as input
  D : Outport
  wires:
  A/1 -> scale/1
  Conversion3/1 -> D/1
  Quantizer/1 -> Saturation/1
  Sampler/1 -> Quantizer/1
  Saturation/1 -> Conversion3/1
  scale/1 -> Sampler/1

== system ddc_bpm_476_066/ADC_16bit_ch2 ==
  A : Inport  OutDataTypeStr=double
  Conversion3 : DataTypeConversion  OutDataTypeStr=fixdt(1,16,2/2^16/1,0/1)  ConvertRealWorld=Stored Integer (SI)  LockScale=on
  Quantizer : Quantizer  QuantizationInterval=1  SampleTime=dt_sim
  Sampler : ZeroOrderHold  SampleTime=1/Fs_adc
  Saturation : Saturate  UpperLimit=65536/2-1  LowerLimit=-65536/2  OutDataTypeStr=Inherit: Inherit via back propagation
  scale : Gain  Gain=2^16/2  SaturateOnIntegerOverflow=on  OutDataTypeStr=Inherit: Same as input  ParamDataTypeStr=Inherit: Same as input
  D : Outport
  wires:
  A/1 -> scale/1
  Conversion3/1 -> D/1
  Quantizer/1 -> Saturation/1
  Sampler/1 -> Quantizer/1
  Saturation/1 -> Conversion3/1
  scale/1 -> Sampler/1

== system ddc_bpm_476_066/ADC_16bit_ch3 ==
  A : Inport  OutDataTypeStr=double
  Conversion3 : DataTypeConversion  OutDataTypeStr=fixdt(1,16,2/2^16/1,0/1)  ConvertRealWorld=Stored Integer (SI)  LockScale=on
  Quantizer : Quantizer  QuantizationInterval=1  SampleTime=dt_sim
  Sampler : ZeroOrderHold  SampleTime=1/Fs_adc
  Saturation : Saturate  UpperLimit=65536/2-1  LowerLimit=-65536/2  OutDataTypeStr=Inherit: Inherit via back propagation
  scale : Gain  Gain=2^16/2  SaturateOnIntegerOverflow=on  OutDataTypeStr=Inherit: Same as input  ParamDataTypeStr=Inherit: Same as input
  D : Outport
  wires:
  A/1 -> scale/1
  Conversion3/1 -> D/1
  Quantizer/1 -> Saturation/1
  Sampler/1 -> Quantizer/1
  Saturation/1 -> Conversion3/1
  scale/1 -> Sampler/1
